simulink model "PV_MPPT_Charging"  (R2022b)
settings: Solver=ode23t  StartTime=0.0  StopTime=10.0  RelTol=1e-3
undefined symbols (not defined in the file or in its folder): Acid, Lead
libraries: spsSeriesRLCBranchLib x3, spsBatteryLib x1, spsDiodeLib x1, spsMosfetLib x1, spsPVArrayLib x1, simulink x1, spspowerguiLib x1
settings Model: Creator=Dell  LastModifiedBy=Budara Abeysinghe
settings SolverCC: AlgebraicLoopSolver=TrustRegion
settings DebuggingCC: UnconnectedInputMsg=warning  UnconnectedOutputMsg=warning  UnconnectedLineMsg=warning  SFMachineParentedDataDiag=warning
settings ModelReferenceCC: EnableRefExpFcnMdlSchedulingChecks=on
settings RTWCC: DLArmComputeVersion=19.05

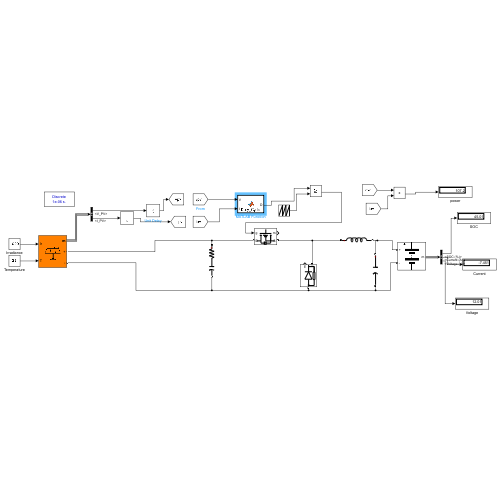
[thumbnail: Simulink's stored preview of the top-level diagram]
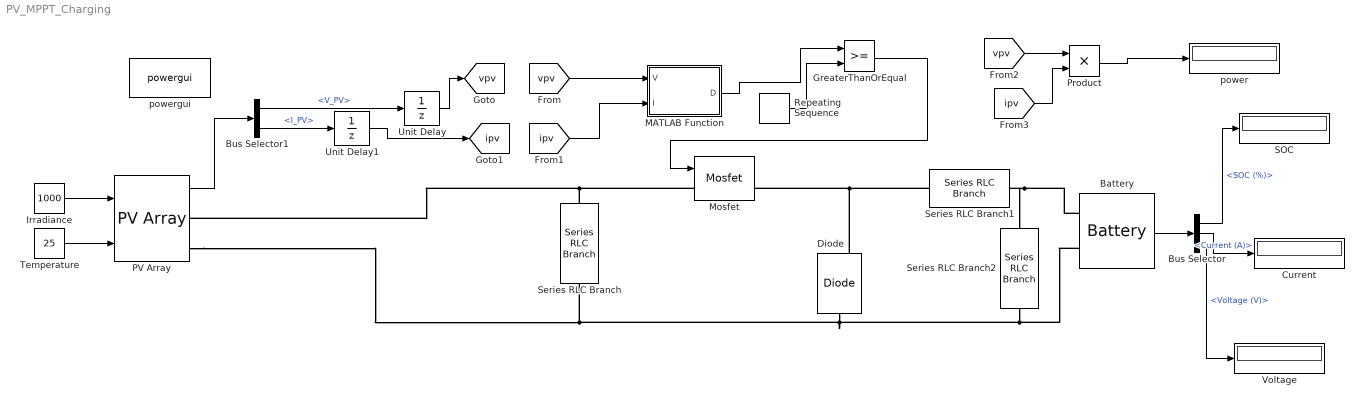
== system PV_MPPT_Charging ==
  Battery : spsBatteryLib/Battery  BatType=Lead-Acid  ShowTempParam=off  ThermalPreset=no  ShowAgeParam=off  NomV=12  NomQ=100  SOC=45  Batt_Tr=1  PresetModel=on  MaxQ=104.1667  MinV=9  FullV=13.0658  Dis_rate=20  R=0.0012  Normal_OP=31.0278  expZone="[12.2171     0.333333]"  current=[6.5 13 32.5]  Units=Time  Tci=20  NomT=20  T2=-30  MaxQ2=4.8  FullV2=7.1  Normal_OP2=5.655  expZone2="[6.58           1]"  Rca=0.6  ti=2000  Dp=0  Neq0=0  Tsim=1e6  Ta1=25  Qeol=5.4*0.9  Reol=0.013333*1.2  Char_age=[2.3478, 3]  Dis_age=[2.3478, 10]  N1=1500  N2=10500  N3=1000  N4=1400  Ta2=45  N5=950
      settings: LibrarySourceBlock=electricdrivelib/Extra Sources/Battery
  Bus Selector : BusSelector  OutputSignals=SOC (%),Current (A),Voltage (V)
  Bus Selector1 : BusSelector  OutputSignals=V_PV,I_PV
  Current : Display
  Diode : spsDiodeLib/Diode  Ron=0.001  Lon=0  Vf=0.8  IC=0  UseSnubber=0  Rs=500  Cs=250e-9  Measurements=on
  GreaterThanOrEqual : RelationalOperator  OutDataTypeStr=boolean  RndMeth=Simplest  InputSameDT=off
  Irradiance : Constant  Value=1000
  MATLAB Function : MATLAB Function  TreatAsAtomicUnit=on
  Mosfet : spsMosfetLib/Mosfet  Ron=0.1  Lon=0  Rd=0.01  Vfd=0  IC=0  Rs=1e5  Cs=inf  Measurements=on
  PV Array : spsPVArrayLib/PV Array  Npar=1  Nser=1  PlotType=array @ 1000 W/m2 & specified temperatures  S_vec="[ 1000  500  100 ]"  Temp_C_vec="[ 45 25  ]"  ModuleName=User-defined  PlotWhenSelected=off  Pm=213.15  Ncell=60  Voc=36.3  Isc=7.84  Vm=29  Im=7.35  beta_Voc_pc=-0.36099  alpha_Isc_pc=0.102  beta_Voc=-0.13104  alpha_Isc=0.0079968  IL=7.8654  I0=2.9273e-10  nI=0.98119  Rsh=313.0553  Rs=0.39381  RobustModel=off  RobustCellTemperature=313.3991  BAL=on  Tc=1e-6  Tfilter=5e-5
  Product : Product
  Repeating Sequence : simulink/Sources/Repeating Sequence  rep_seq_t=[0 0.0002]  rep_seq_y=[0 1]
  SOC : Display
  Series RLC Branch : spsSeriesRLCBranchLib/Series RLC Branch  LConnTagsString=__new0  RConnTagsString=__new0  BranchType=RC  Resistance=0.001  Inductance=1e-3  SetiL0=off  InitialCurrent=0  Capacitance=1000e-6  Setx0=off  InitialVoltage=0  Measurements=None
  Series RLC Branch1 : spsSeriesRLCBranchLib/Series RLC Branch  LConnTagsString=__new0  RConnTagsString=__new0  BranchType=L  Resistance=1  Inductance=0.8653e-3  SetiL0=off  InitialCurrent=0  Capacitance=1e-6  Setx0=off  InitialVoltage=0  Measurements=None
  Series RLC Branch2 : spsSeriesRLCBranchLib/Series RLC Branch  LConnTagsString=__new0  RConnTagsString=__new0  BranchType=C  Resistance=1  Inductance=369.79e-6  SetiL0=off  InitialCurrent=0  Capacitance=369.79e-6  Setx0=off  InitialVoltage=0  Measurements=None
  Temperature : Constant  Value=25
  Unit Delay : UnitDelay  SampleTime=1e-4  HasFrameUpgradeWarning=on
  Unit Delay1 : UnitDelay  SampleTime=1e-4  HasFrameUpgradeWarning=on
  Voltage : Display
  power : Display
  powergui : spspowerguiLib/powergui  Priority=1  SimulationMode=Discrete  SampleTime=1e-6  frequency=60  Iterations=50  frequencyindice=0  Pbase=100e6  ErrMax=1e-4  UnitsV=kV  UnitsW=MW  buscounter=0  FunctionMessages=off  echomessages=off  EnableUseOfTLC=off  CurrentSourceSwitches=off  DisableSnubberDevices=off  DisableRonSwitches=off  DisableVfSwitches=off  DisplayEquations=off  AutomaticDiscreteSolvers=off  SolverType=Tustin/Backward Euler (TBE)  Interpol=off  ExternalGateDelay=off  methode=off  Ts=100  x0status=blocks  SPID=on  SwTol=0  HookPort=off  NonlinearTolerance=1e-4  nMaxIteration=100  ContinueOnMaxIteration=off  RestoreLinks=warning  ResistiveCurrentMeasurement=off  Frange=[0:2:500]  Ylog=off  Xlog=on  ShowGrid=off  save=off  variable=ZData  structure=0  ZoomFFT=off  StartTime=0.0  cycles=1  DisplayStyle=1  fundamental=60  FreqAxis=off  MaxFrequency=1000  frequencyindicesteady=1  RmsSteady=1  display=off
  tag scope: ipv=global, vpv=global
  wires:
  Irradiance/1 -> PV Array/1
  Temperature/1 -> PV Array/2
  Battery/1 -> Bus Selector/1
  Bus Selector/1 -> SOC/1  "<SOC (%)>"
  Bus Selector/3 -> Voltage/1  "<Voltage (V)>"
  Bus Selector/2 -> Current/1  "<Current (A)>"
  PV Array/1 -> Bus Selector1/1
  Bus Selector1/1 -> Unit Delay/1  "<V_PV>"
  Bus Selector1/2 -> Unit Delay1/1  "<I_PV>"
  Unit Delay/1 -> [vpv]
  Unit Delay1/1 -> [ipv]
  [vpv] -> MATLAB Function/1(V)
  [ipv] -> MATLAB Function/2(I)
  MATLAB Function/1(D) -> GreaterThanOrEqual/1
  Repeating Sequence/1 -> GreaterThanOrEqual/2
  GreaterThanOrEqual/1 -> Mosfet/1
  [vpv] -> Product/1
  [ipv] -> Product/2
  Product/1 -> power/1
  connections:
  Series RLC Branch/LConn1 -- Mosfet/LConn1 -- PV Array/RConn1
  PV Array/RConn2 -- Battery/LConn2 -- Series RLC Branch2/RConn1 -- Diode/LConn1 -- Series RLC Branch/RConn1
  Diode/RConn1 -- Series RLC Branch1/LConn1 -- Mosfet/RConn1
  Battery/LConn1 -- Series RLC Branch2/LConn1 -- Series RLC Branch1/RConn1

== matlab function PV_MPPT_Charging/MATLAB Function ==
  data: V input; D output; I input
function D = Duty_Cycle(V,I)
Dmax = 0.95;
Dmin = 0;
Dinit = 0.95;
DelD = 0.0001;
persistent Vold Pold Dold;

datatype = 'double' ;

if isempty(Vold)
    Vold = 0;
    Pold = 0;
    Dold = Dinit;
end

P = V*I;
dV = V-Vold;
dP = P - Pold;
if dP ~= 0;
    if dP < 0;
        if dV<0
            D = Dold-DelD;
        else
            D = Dold - DelD;
        end
    else 
        if dV < 0
            D = Dold + DelD;
        else 
            D = Dold - DelD;
        end
    end
else D = Dold;
end

if D >= Dmax || D < Dmin 
    D = Dold;
end
Dold = D;
Vold = V;
Pold = P;
